simulink model "EngDem_TrqLimCoord"  (R2018a)
settings: configuration reference "cs_ert" (kept outside this file)
model workspace (MAT data in the model file):
  EngDem_TrqLimCoord_DT = 10
values from neighbouring files (symbols this model uses):
  EngDem_facAdj_C = 1.0    [EngDem_TrqLimCoord.sldd]
  EngDem_facAdjMax_C = 1.0    [EngDem_TrqLimCoord.sldd]
  EngDem_facAdjMin_C = 1.0    [EngDem_TrqLimCoord.sldd]
  EngDem_facDvolPT1_C = 50.0    [EngDem_TrqLimCoord.sldd]
  EngDem_facResFlowPT1_C = 50.0    [EngDem_TrqLimCoord.sldd]
  EngDem_RmpLimErrNeg_C = 50.0    [EngDem_TrqLimCoord.sldd]
  EngDem_RmpLimErrPos_C = 50.0    [EngDem_TrqLimCoord.sldd]
  EngDem_trqLimErr1_CUR : value not decoded    [EngDem_TrqLimCoord.sldd]
  EngDem_trqLimErr1_CURX : value not decoded    [EngDem_TrqLimCoord.sldd]
  EngDem_trqLimErr2_CUR : value not decoded    [EngDem_TrqLimCoord.sldd]
  EngDem_trqLimErr2_CURX : value not decoded    [EngDem_TrqLimCoord.sldd]
  EngDem_trqLimErr3_CUR : value not decoded    [EngDem_TrqLimCoord.sldd]
  EngDem_trqLimErr3_CURX : value not decoded    [EngDem_TrqLimCoord.sldd]
  EngDem_trqLimErr4_CUR : value not decoded    [EngDem_TrqLimCoord.sldd]
  EngDem_trqLimErr4_CURX : value not decoded    [EngDem_TrqLimCoord.sldd]
  EngDem_TrqLimErrRmpNeg_C = 50.0    [EngDem_TrqLimCoord.sldd]
  EngDem_TrqLimErrRmpPos_C = 100.0    [EngDem_TrqLimCoord.sldd]
  EngDem_trqLimPDiff_CUR : value not decoded    [EngDem_TrqLimCoord.sldd]
  EngDem_trqLimPDiff_CURX : value not decoded    [EngDem_TrqLimCoord.sldd]
undefined symbols (not defined in the file or in its folder): CEngDsT_tTransf_CURX, TRQ_MAX
libraries: sllib x4, simulink x2
settings Model: DataDictionary=EngDem_TrqLimCoord.sldd  Creator=zhoutinglin  LastModifiedBy=zhoutinglin

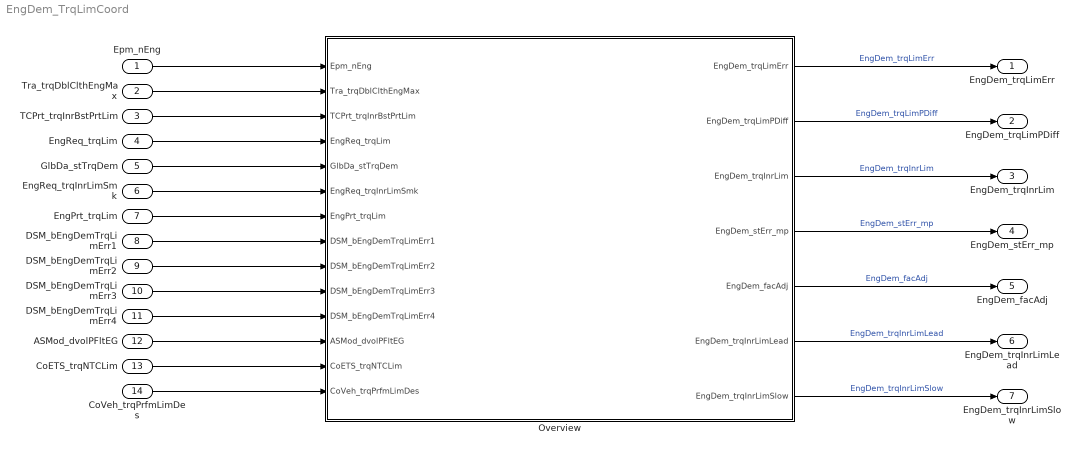
== system EngDem_TrqLimCoord ==
  Epm_nEng : Inport  Description=Engine speed  OutMin=0  OutMax=6000  OutDataTypeStr=ERPM  Unit=rpm  PortDimensions=[1 1]
  Tra_trqDblClthEngMax : Inport  Description=Application parameter for minimum torque of systemdegratation Nm  Port=2  OutMin=-3000  OutMax=3000  OutDataTypeStr=Torq  Unit=Nm  PortDimensions=[1 1]
  TCPrt_trqInrBstPrtLim : Inport  Description=Torque limitation from VGT Nm  Port=3  OutMin=-3276.8  OutMax=3276.7  OutDataTypeStr=Torq  Unit=Nm  PortDimensions=[1 1]
  EngReq_trqLim : Inport  Description=Resulting limiting torque from engine specifications  Port=4  OutMin=-3276.8  OutMax=3276.7  OutDataTypeStr=Torq  Unit=Nm  PortDimensions=[1 1]
  GlbDa_stTrqDem : Inport  Description=contains highest prior function with torque demand  Port=5  OutMin=0  OutMax=4294967295  OutDataTypeStr=State4  PortDimensions=[1 1]
  EngReq_trqInrLimSmk : Inport  Description=Limiting torque smoke limit  Port=6  OutMin=-3276.8  OutMax=3276.7  OutDataTypeStr=Torq  Unit=Nm  PortDimensions=[1 1]
  EngPrt_trqLim : Inport  Description=Limitation torque for engine mechanic protection by torque limitation (as inner engine torque)  Port=7  OutMin=-3276.8  OutMax=3276.7  OutDataTypeStr=Torq  Unit=Nm  PortDimensions=[1 1]
  DSM_bEngDemTrqLimErr1 : Inport  Description=FId for Engine demand Torque Limitation due to System error  Port=8  OutMin=0  OutMax=1  OutDataTypeStr=boolean  PortDimensions=[1 1]
  DSM_bEngDemTrqLimErr2 : Inport  Description=FId for Engine demand Torque Limitation due to System error  Port=9  OutMin=0  OutMax=1  OutDataTypeStr=boolean  PortDimensions=[1 1]
  DSM_bEngDemTrqLimErr3 : Inport  Description=FId for Engine demand Torque Limitation due to System error  Port=10  OutMin=0  OutMax=1  OutDataTypeStr=boolean  PortDimensions=[1 1]
  DSM_bEngDemTrqLimErr4 : Inport  Description=FId for Engine demand Torque Limitation due to System error  Port=11  OutMin=0  OutMax=1  OutDataTypeStr=boolean  PortDimensions=[1 1]
  ASMod_dvolPFltEG : Inport  Description=Calculated exhaust-gas volume flow in the particulate filter  Port=12  OutMin=0  OutMax=100  OutDataTypeStr=vFlow_m3ph  Unit=m^3/h  PortDimensions=[1 1]
  CoETS_trqNTCLim : Inport  Description=NTC torque limitation (0 in braking, ramped to max in braked to fired  Port=13  OutMin=0  OutMax=1000  OutDataTypeStr=Torq  Unit=Nm  PortDimensions=[1 1]
  CoVeh_trqPrfmLimDes : Inport  Description=Torque limitation from performence limiter  Port=14  OutMin=-3000  OutMax=3276.7  OutDataTypeStr=Torq  Unit=Nm  PortDimensions=[1 1]
  Overview : Subsystem
  EngDem_trqLimErr : Outport
  EngDem_trqLimPDiff : Outport  Port=2
  EngDem_trqInrLim : Outport  Port=3
  EngDem_stErr_mp : Outport  Port=4
  EngDem_facAdj : Outport  Port=5
  EngDem_trqInrLimLead : Outport  Port=6
  EngDem_trqInrLimSlow : Outport  Port=7
  wires:
  Epm_nEng/1 -> Overview/1(Epm_nEng)
  Tra_trqDblClthEngMax/1 -> Overview/2(Tra_trqDblClthEngMax)
  TCPrt_trqInrBstPrtLim/1 -> Overview/3(TCPrt_trqInrBstPrtLim)
  EngReq_trqLim/1 -> Overview/4(EngReq_trqLim)
  GlbDa_stTrqDem/1 -> Overview/5(GlbDa_stTrqDem)
  EngReq_trqInrLimSmk/1 -> Overview/6(EngReq_trqInrLimSmk)
  EngPrt_trqLim/1 -> Overview/7(EngPrt_trqLim)
  DSM_bEngDemTrqLimErr1/1 -> Overview/8(DSM_bEngDemTrqLimErr1)
  DSM_bEngDemTrqLimErr2/1 -> Overview/9(DSM_bEngDemTrqLimErr2)
  DSM_bEngDemTrqLimErr3/1 -> Overview/10(DSM_bEngDemTrqLimErr3)
  DSM_bEngDemTrqLimErr4/1 -> Overview/11(DSM_bEngDemTrqLimErr4)
  ASMod_dvolPFltEG/1 -> Overview/12(ASMod_dvolPFltEG)
  CoETS_trqNTCLim/1 -> Overview/13(CoETS_trqNTCLim)
  CoVeh_trqPrfmLimDes/1 -> Overview/14(CoVeh_trqPrfmLimDes)
  Overview/1(EngDem_trqLimErr) -> EngDem_trqLimErr/1  "EngDem_trqLimErr"
  Overview/2(EngDem_trqLimPDiff) -> EngDem_trqLimPDiff/1  "EngDem_trqLimPDiff"
  Overview/3(EngDem_trqInrLim) -> EngDem_trqInrLim/1  "EngDem_trqInrLim"
  Overview/4(EngDem_stErr_mp) -> EngDem_stErr_mp/1  "EngDem_stErr_mp"
  Overview/5(EngDem_facAdj) -> EngDem_facAdj/1  "EngDem_facAdj"
  Overview/6(EngDem_trqInrLimLead) -> EngDem_trqInrLimLead/1  "EngDem_trqInrLimLead"
  Overview/7(EngDem_trqInrLimSlow) -> EngDem_trqInrLimSlow/1  "EngDem_trqInrLimSlow"

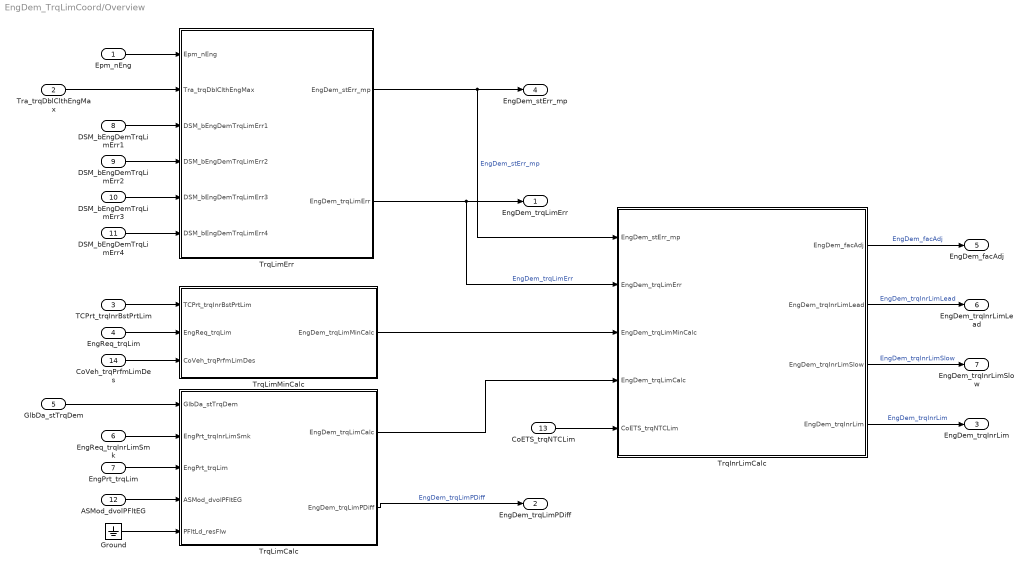
== system EngDem_TrqLimCoord/Overview ==
  Epm_nEng : Inport  Tag=rpm  Description=Engine speed  OutMin=0  OutMax=6000
  Tra_trqDblClthEngMax : Inport  Tag=Nm  Description=Application parameter for minimum torque of systemdegratation Nm  Port=2  OutMin=-3000  OutMax=3000
  TCPrt_trqInrBstPrtLim : Inport  Tag=Nm  Description=Torque limitation from VGT Nm  Port=3  OutMin=-3276.8  OutMax=3276.7
  EngReq_trqLim : Inport  Tag=Nm  Description=Resulting limiting torque from engine specifications  Port=4  OutMin=-3276.8  OutMax=3276.7
  GlbDa_stTrqDem : Inport  Description=contains highest prior function with torque demand  Port=5  OutMin=0  OutMax=4294967295
  EngReq_trqInrLimSmk : Inport  Tag=Nm  Description=Limiting torque smoke limit  Port=6  OutMin=-3276.8  OutMax=3276.7
  EngPrt_trqLim : Inport  Tag=Nm  Description=Limitation torque for engine mechanic protection by torque limitation (as inner engine torque)  Port=7  OutMin=-3276.8  OutMax=3276.7
  DSM_bEngDemTrqLimErr1 : Inport  Description=FId for Engine demand Torque Limitation due to System error  Port=8  OutMin=0  OutMax=1  OutDataTypeStr=boolean
  DSM_bEngDemTrqLimErr2 : Inport  Description=FId for Engine demand Torque Limitation due to System error  Port=9  OutMin=0  OutMax=1  OutDataTypeStr=boolean
  DSM_bEngDemTrqLimErr3 : Inport  Description=FId for Engine demand Torque Limitation due to System error  Port=10  OutMin=0  OutMax=1  OutDataTypeStr=boolean
  DSM_bEngDemTrqLimErr4 : Inport  Description=FId for Engine demand Torque Limitation due to System error  Port=11  OutMin=0  OutMax=1  OutDataTypeStr=boolean
  ASMod_dvolPFltEG : Inport  Tag=m^3/h  Description=Calculated exhaust-gas volume flow in the particulate filter  Port=12  OutMin=0  OutMax=100
  CoETS_trqNTCLim : Inport  Tag=Nm  Description=NTC torque limitation (0 in braking, ramped to max in braked to fired  Port=13  OutMin=0  OutMax=1000
  CoVeh_trqPrfmLimDes : Inport  Tag=Nm  Description=Torque limitation from performence limiter  Port=14  OutMin=-3000  OutMax=3276.7
  Ground : Ground
  TrqInrLimCalc : Subsystem
  TrqLimCalc : Subsystem  RTWFcnName=TrqLimCalc_Co  RTWFileName=TrqLimCalc
      settings: RTWSystemCode=Nonreusable function  RTWFcnNameOpts=User specified  RTWFileNameOpts=User specified
  TrqLimErr : Subsystem  RTWFcnName=TrqLimErr_Co  RTWFileName=TrqLimErr
      settings: RTWSystemCode=Nonreusable function  RTWFcnNameOpts=User specified  RTWFileNameOpts=User specified
  TrqLimMinCalc : Subsystem  RTWFcnName=TrqLimMinCalc_Co  RTWFileName=TrqLimMinCalc
      settings: RTWSystemCode=Nonreusable function  RTWFcnNameOpts=User specified  RTWFileNameOpts=User specified
  EngDem_trqLimErr : Outport  Tag=Nm  Description=Substitute limiting torque in the event of an error  OutMin=-3276.8  OutMax=3276.7
  EngDem_trqLimPDiff : Outport  Tag=Nm  Description=Limiting torque due to exhaust gas back-pressure  Port=2  OutMin=-3276.8  OutMax=3276.7
  EngDem_trqInrLim : Outport  Tag=Nm  Description=Resulting limiting torque (inner engine torque)  Port=3  OutMin=-3276.8  OutMax=3276.7
  EngDem_stErr_mp : Outport  Description=Status of the limitation FIDs  Port=4  OutMin=0  OutMax=1  OutDataTypeStr=boolean
  EngDem_facAdj : Outport  Description=EEPROM adjustment value for correction of the limiting torque  Port=5  OutMin=-10  OutMax=10
  EngDem_trqInrLimLead : Outport  Tag=Nm  Description=inner engine limted lead torque  Port=6  OutMin=-3276.8  OutMax=3276.7
  EngDem_trqInrLimSlow : Outport  Tag=Nm  Description=inner engine limted torque for Slow Path  Port=7  OutMin=-3276.8  OutMax=3276.7
  wires:
  Epm_nEng/1 -> TrqLimErr/1(Epm_nEng)
  TrqLimCalc/1(EngDem_trqLimCalc) -> TrqInrLimCalc/4(EngDem_trqLimCalc)
  CoETS_trqNTCLim/1 -> TrqInrLimCalc/5(CoETS_trqNTCLim)
  TrqInrLimCalc/2(EngDem_trqInrLimLead) -> EngDem_trqInrLimLead/1  "EngDem_trqInrLimLead"
  TrqLimCalc/2(EngDem_trqLimPDiff) -> EngDem_trqLimPDiff/1  "EngDem_trqLimPDiff"
  CoVeh_trqPrfmLimDes/1 -> TrqLimMinCalc/3(CoVeh_trqPrfmLimDes)
  DSM_bEngDemTrqLimErr3/1 -> TrqLimErr/5(DSM_bEngDemTrqLimErr3)
  Tra_trqDblClthEngMax/1 -> TrqLimErr/2(Tra_trqDblClthEngMax)
  TrqLimErr/2(EngDem_trqLimErr) -> EngDem_trqLimErr/1, TrqInrLimCalc/2(EngDem_trqLimErr)  "EngDem_trqLimErr"
  DSM_bEngDemTrqLimErr2/1 -> TrqLimErr/4(DSM_bEngDemTrqLimErr2)
  TrqLimMinCalc/1(EngDem_trqLimMinCalc) -> TrqInrLimCalc/3(EngDem_trqLimMinCalc)
  TrqInrLimCalc/3(EngDem_trqInrLimSlow) -> EngDem_trqInrLimSlow/1  "EngDem_trqInrLimSlow"
  TrqInrLimCalc/4(EngDem_trqInrLim) -> EngDem_trqInrLim/1  "EngDem_trqInrLim"
  DSM_bEngDemTrqLimErr4/1 -> TrqLimErr/6(DSM_bEngDemTrqLimErr4)
  TrqLimErr/1(EngDem_stErr_mp) -> EngDem_stErr_mp/1, TrqInrLimCalc/1(EngDem_stErr_mp)  "EngDem_stErr_mp"
  EngReq_trqLim/1 -> TrqLimMinCalc/2(EngReq_trqLim)
  EngPrt_trqLim/1 -> TrqLimCalc/3(EngPrt_trqLim)
  DSM_bEngDemTrqLimErr1/1 -> TrqLimErr/3(DSM_bEngDemTrqLimErr1)
  GlbDa_stTrqDem/1 -> TrqLimCalc/1(GlbDa_stTrqDem)
  TCPrt_trqInrBstPrtLim/1 -> TrqLimMinCalc/1(TCPrt_trqInrBstPrtLim)
  EngReq_trqInrLimSmk/1 -> TrqLimCalc/2(EngPrt_trqInrLimSmk)
  Ground/1 -> TrqLimCalc/5(PFltLd_resFlw)
  TrqInrLimCalc/1(EngDem_facAdj) -> EngDem_facAdj/1  "EngDem_facAdj"
  ASMod_dvolPFltEG/1 -> TrqLimCalc/4(ASMod_dvolPFltEG)

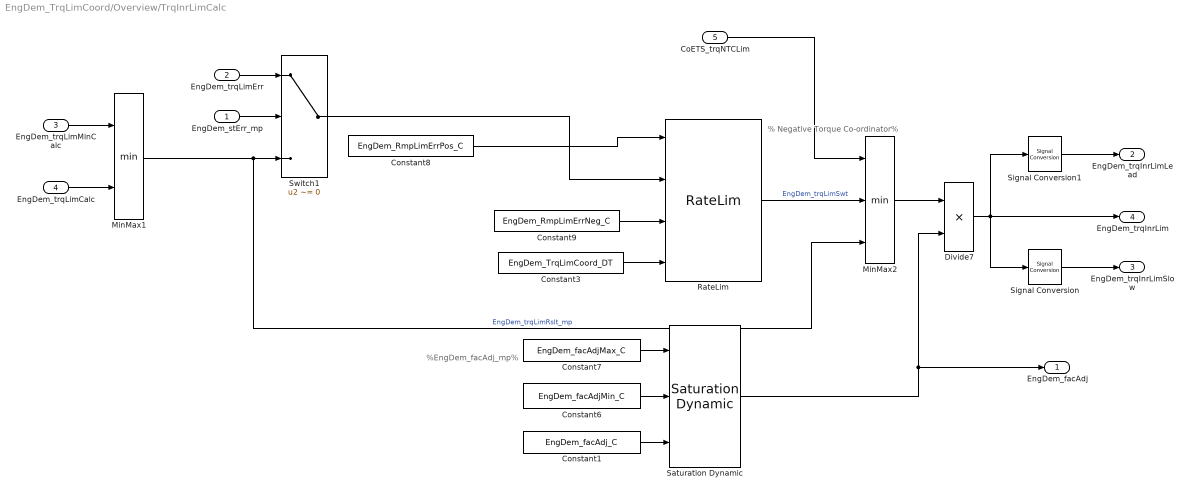
== system EngDem_TrqLimCoord/Overview/TrqInrLimCalc ==
  note: % Negative Torque Co-ordinator%
  note: %EngDem_facAdj_mp%
  EngDem_stErr_mp : Inport
  EngDem_trqLimErr : Inport  Port=2
  EngDem_trqLimMinCalc : Inport  Port=3
  EngDem_trqLimCalc : Inport  Port=4
  CoETS_trqNTCLim : Inport  Tag=Nm  Description=NTC torque limitation (0 in braking, ramped to max in braked to fired  Port=5
  Constant1 : Constant  Value=EngDem_facAdj_C
  Constant3 : Constant  Value=EngDem_TrqLimCoord_DT  OutDataTypeStr=Inherit: Inherit via back propagation
  Constant6 : Constant  Value=EngDem_facAdjMin_C
  Constant7 : Constant  Value=EngDem_facAdjMax_C
  Constant8 : Constant  Value=EngDem_RmpLimErrPos_C
  Constant9 : Constant  Value=EngDem_RmpLimErrNeg_C
  Divide7 : Product  Inputs=**  OutDataTypeStr=Inherit: Inherit via back propagation
  MinMax1 : MinMax  Inputs=2  InputSameDT=on
  MinMax2 : MinMax  Inputs=3  InputSameDT=on
  RateLim : sllib/RateLim
      settings: SourceProductName=sllib
  Saturation Dynamic : simulink/Discontinuities/Saturation Dynamic  OutMin=[]  OutMax=[]  OutDataTypeStr=Inherit: Same as second input  OutDataType=fixdt(1, 16)  OutScaling=2^-10  DoSatur=off
  Signal Conversion : SignalConversion  OverrideOpt=off
  Signal Conversion1 : SignalConversion  OverrideOpt=off
  Switch1 : Switch  Criteria=u2 ~= 0  InputSameDT=on
  EngDem_facAdj : Outport
  EngDem_trqInrLimLead : Outport  Port=2
  EngDem_trqInrLimSlow : Outport  Port=3
  EngDem_trqInrLim : Outport  Port=4
  wires:
  MinMax2/1 -> Divide7/1
  MinMax1/1 -> MinMax2/3, Switch1/3  "EngDem_trqLimRslt_mp"
  EngDem_trqLimCalc/1 -> MinMax1/2
  Constant1/1 -> Saturation Dynamic/3
  Constant6/1 -> Saturation Dynamic/2
  CoETS_trqNTCLim/1 -> MinMax2/1
  EngDem_trqLimMinCalc/1 -> MinMax1/1
  Constant7/1 -> Saturation Dynamic/1
  Saturation Dynamic/1 -> EngDem_facAdj/1, Divide7/2
  RateLim/1 -> MinMax2/2  "EngDem_trqLimSwt"
  Constant9/1 -> RateLim/3
  Constant8/1 -> RateLim/1
  Switch1/1 -> RateLim/2
  EngDem_trqLimErr/1 -> Switch1/1
  EngDem_stErr_mp/1 -> Switch1/2
  Constant3/1 -> RateLim/4
  Divide7/1 -> EngDem_trqInrLim/1, Signal Conversion/1, Signal Conversion1/1
  Signal Conversion1/1 -> EngDem_trqInrLimLead/1
  Signal Conversion/1 -> EngDem_trqInrLimSlow/1

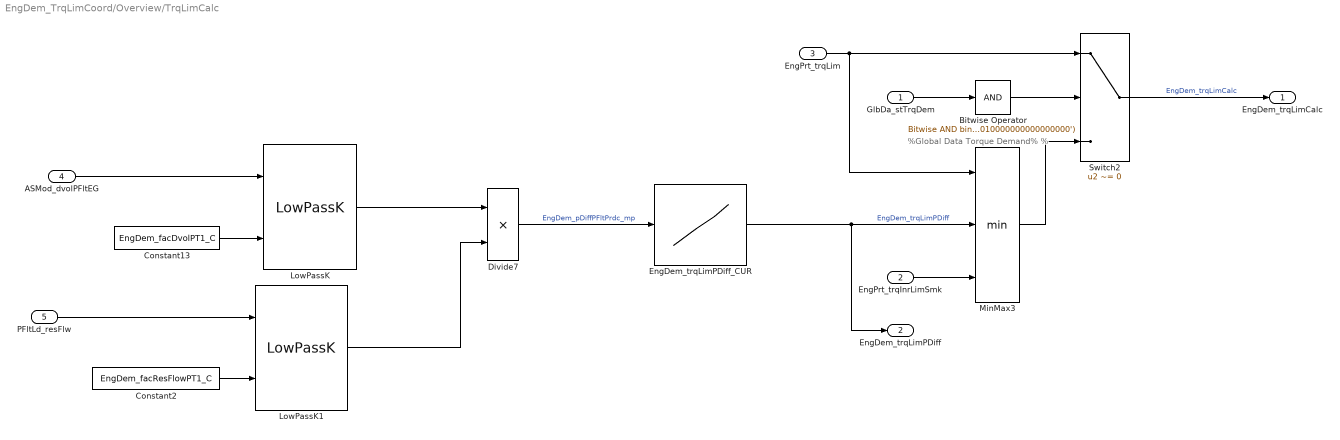
== system EngDem_TrqLimCoord/Overview/TrqLimCalc ==
  note: %Global Data Torque Demand% %
  GlbDa_stTrqDem : Inport
  EngPrt_trqInrLimSmk : Inport  Port=2
  EngPrt_trqLim : Inport  Port=3
  ASMod_dvolPFltEG : Inport  Tag=m^2/h  Description=Calculated exhaust-gas volume flow in the particulate filter  Port=4
  PFltLd_resFlw : Inport  Tag=kPa/(m^2/h)  Description=Flow resistance of the particulate filter  Port=5
  Bitwise Operator : simulink/Logic and Bit Operations/Bitwise Operator  logicop=AND  UseBitMask=on  BitMask=bin2dec('00000000000000010000000000000000')  BitMaskRealWorld=Stored Integer
  Constant13 : Constant  Value=EngDem_facDvolPT1_C
  Constant2 : Constant  Value=EngDem_facResFlowPT1_C
  Divide7 : Product  Inputs=**  OutDataTypeStr=Inherit: Inherit via back propagation
  EngDem_trqLimPDiff_CUR : Lookup_n-D  DialogController=Simulink.DDGSource  NumberOfTableDimensions=1  BreakpointsForDimension1=EngDem_trqLimPDiff_CURX  BreakpointsForDimension2=CEngDsT_tTransf_CURX  IndexSearchMethod=Linear search  BeginIndexSearchUsingPreviousIndexResult=on  Table=EngDem_trqLimPDiff_CUR  ExtrapMethod=Clip  UseLastTableValue=on  InternalRulePriority=Speed  OutDataTypeStr=Inherit: Inherit via back propagation  SaturateOnIntegerOverflow=on
  LowPassK : sllib/LowPassK
      settings: SourceProductName=sllib
  LowPassK1 : sllib/LowPassK
      settings: SourceProductName=sllib
  MinMax3 : MinMax  Inputs=3  InputSameDT=on
  Switch2 : Switch  Criteria=u2 ~= 0  InputSameDT=on
  EngDem_trqLimCalc : Outport
  EngDem_trqLimPDiff : Outport  Port=2
  wires:
  GlbDa_stTrqDem/1 -> Bitwise Operator/1
  EngPrt_trqLim/1 -> MinMax3/1, Switch2/1
  MinMax3/1 -> Switch2/3
  EngDem_trqLimPDiff_CUR/1 -> EngDem_trqLimPDiff/1, MinMax3/2  "EngDem_trqLimPDiff"
  Divide7/1 -> EngDem_trqLimPDiff_CUR/1  "EngDem_pDiffPFltPrdc_mp"
  ASMod_dvolPFltEG/1 -> LowPassK/1
  EngPrt_trqInrLimSmk/1 -> MinMax3/3
  Switch2/1 -> EngDem_trqLimCalc/1  "EngDem_trqLimCalc"
  Constant13/1 -> LowPassK/2
  Bitwise Operator/1 -> Switch2/2
  LowPassK1/1 -> Divide7/2
  LowPassK/1 -> Divide7/1
  Constant2/1 -> LowPassK1/2
  PFltLd_resFlw/1 -> LowPassK1/1

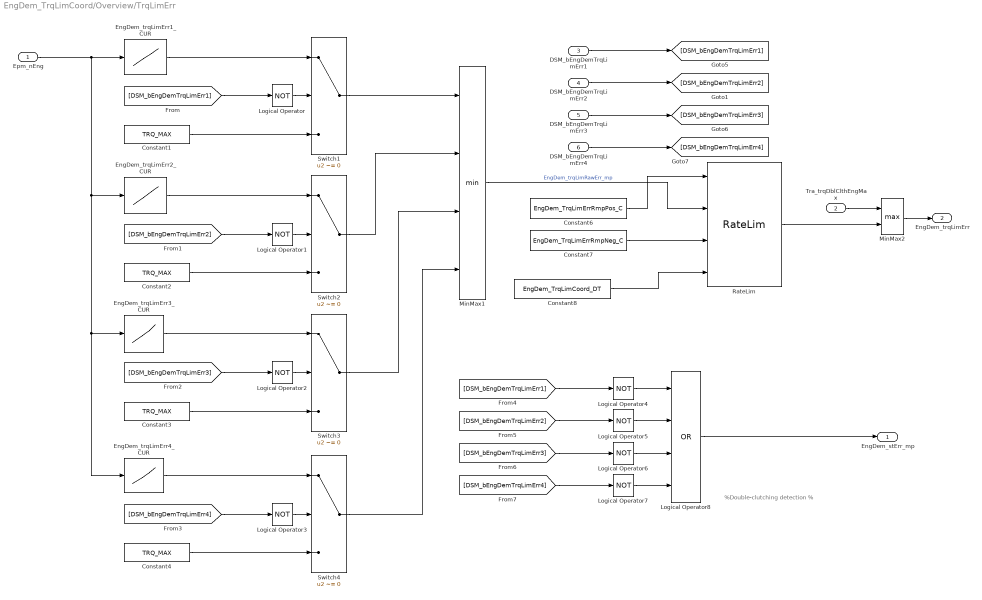
== system EngDem_TrqLimCoord/Overview/TrqLimErr ==
  note: %Double-clutching detection %
  Epm_nEng : Inport  Description=Engine speed
  Tra_trqDblClthEngMax : Inport  Port=2
  DSM_bEngDemTrqLimErr1 : Inport  Description=status of FId_EngDemTrqLimErr1  Port=3  OutMin=0  OutMax=1  OutDataTypeStr=boolean
  DSM_bEngDemTrqLimErr2 : Inport  Description=status of FId_EngDemTrqLimErr2  Port=4  OutMin=0  OutMax=1  OutDataTypeStr=boolean
  DSM_bEngDemTrqLimErr3 : Inport  Description=status of FId_EngDemTrqLimErr3  Port=5  OutMin=0  OutMax=1  OutDataTypeStr=boolean
  DSM_bEngDemTrqLimErr4 : Inport  Description=status of FId_EngDemTrqLimErr4  Port=6  OutMin=0  OutMax=1  OutDataTypeStr=boolean
  Constant{1..4} (4 alike) : Constant  Value=TRQ_MAX
  Constant6 : Constant  Value=EngDem_TrqLimErrRmpPos_C
  Constant7 : Constant  Value=EngDem_TrqLimErrRmpNeg_C
  Constant8 : Constant  Value=EngDem_TrqLimCoord_DT  OutDataTypeStr=Inherit: Inherit via back propagation
  EngDem_trqLimErr1_CUR : Lookup_n-D  DialogController=Simulink.DDGSource  NumberOfTableDimensions=1  BreakpointsForDimension1=EngDem_trqLimErr1_CURX  BreakpointsForDimension2=CEngDsT_tTransf_CURX  IndexSearchMethod=Linear search  BeginIndexSearchUsingPreviousIndexResult=on  Table=EngDem_trqLimErr1_CUR  ExtrapMethod=Clip  UseLastTableValue=on  InternalRulePriority=Speed  OutDataTypeStr=Inherit: Inherit via back propagation  SaturateOnIntegerOverflow=on
  EngDem_trqLimErr2_CUR : Lookup_n-D  DialogController=Simulink.DDGSource  NumberOfTableDimensions=1  BreakpointsForDimension1=EngDem_trqLimErr2_CURX  BreakpointsForDimension2=CEngDsT_tTransf_CURX  IndexSearchMethod=Linear search  BeginIndexSearchUsingPreviousIndexResult=on  Table=EngDem_trqLimErr2_CUR  ExtrapMethod=Clip  UseLastTableValue=on  InternalRulePriority=Speed  OutDataTypeStr=Inherit: Inherit via back propagation  SaturateOnIntegerOverflow=on
  EngDem_trqLimErr3_CUR : Lookup_n-D  DialogController=Simulink.DDGSource  NumberOfTableDimensions=1  BreakpointsForDimension1=EngDem_trqLimErr3_CURX  BreakpointsForDimension2=CEngDsT_tTransf_CURX  IndexSearchMethod=Linear search  BeginIndexSearchUsingPreviousIndexResult=on  Table=EngDem_trqLimErr3_CUR  ExtrapMethod=Clip  UseLastTableValue=on  InternalRulePriority=Speed  OutDataTypeStr=Inherit: Inherit via back propagation  SaturateOnIntegerOverflow=on
  EngDem_trqLimErr4_CUR : Lookup_n-D  DialogController=Simulink.DDGSource  NumberOfTableDimensions=1  BreakpointsForDimension1=EngDem_trqLimErr4_CURX  BreakpointsForDimension2=CEngDsT_tTransf_CURX  IndexSearchMethod=Linear search  BeginIndexSearchUsingPreviousIndexResult=on  Table=EngDem_trqLimErr4_CUR  ExtrapMethod=Clip  UseLastTableValue=on  InternalRulePriority=Speed  OutDataTypeStr=Inherit: Inherit via back propagation  SaturateOnIntegerOverflow=on
  Logical Operator{,1..7} (8 alike) : Logic  Operator=NOT  AllPortsSameDT=off  OutDataTypeStr=boolean
  Logical Operator8 : Logic  Operator=OR  Inputs=4  AllPortsSameDT=off  OutDataTypeStr=boolean
  MinMax1 : MinMax  Inputs=4  InputSameDT=on
  MinMax2 : MinMax  Function=max  Inputs=2  InputSameDT=on
  RateLim : sllib/RateLim
      settings: SourceProductName=sllib
  Switch{1..4} (4 alike) : Switch  Criteria=u2 ~= 0  InputSameDT=on
  EngDem_stErr_mp : Outport
  EngDem_trqLimErr : Outport  Port=2
  wires:
  MinMax1/1 -> RateLim/2  "EngDem_trqLimRawErr_mp"
  Switch1/1 -> MinMax1/1
  Logical Operator/1 -> Switch1/2
  [DSM_bEngDemTrqLimErr1] -> Logical Operator/1
  EngDem_trqLimErr1_CUR/1 -> Switch1/1
  Logical Operator1/1 -> Switch2/2
  [DSM_bEngDemTrqLimErr2] -> Logical Operator1/1
  EngDem_trqLimErr2_CUR/1 -> Switch2/1
  Switch2/1 -> MinMax1/2
  Logical Operator2/1 -> Switch3/2
  [DSM_bEngDemTrqLimErr3] -> Logical Operator2/1
  EngDem_trqLimErr3_CUR/1 -> Switch3/1
  Switch3/1 -> MinMax1/3
  Logical Operator3/1 -> Switch4/2
  [DSM_bEngDemTrqLimErr4] -> Logical Operator3/1
  EngDem_trqLimErr4_CUR/1 -> Switch4/1
  Switch4/1 -> MinMax1/4
  Epm_nEng/1 -> EngDem_trqLimErr4_CUR/1, EngDem_trqLimErr3_CUR/1, EngDem_trqLimErr2_CUR/1, EngDem_trqLimErr1_CUR/1
  Tra_trqDblClthEngMax/1 -> MinMax2/1
  Logical Operator4/1 -> Logical Operator8/1
  Logical Operator5/1 -> Logical Operator8/2
  Logical Operator6/1 -> Logical Operator8/3
  Logical Operator7/1 -> Logical Operator8/4
  Constant6/1 -> RateLim/1
  Constant7/1 -> RateLim/3
  RateLim/1 -> MinMax2/2
  Logical Operator8/1 -> EngDem_stErr_mp/1
  Constant1/1 -> Switch1/3
  Constant2/1 -> Switch2/3
  Constant3/1 -> Switch3/3
  Constant4/1 -> Switch4/3
  DSM_bEngDemTrqLimErr1/1 -> [DSM_bEngDemTrqLimErr1]
  DSM_bEngDemTrqLimErr2/1 -> [DSM_bEngDemTrqLimErr2]
  DSM_bEngDemTrqLimErr3/1 -> [DSM_bEngDemTrqLimErr3]
  DSM_bEngDemTrqLimErr4/1 -> [DSM_bEngDemTrqLimErr4]
  [DSM_bEngDemTrqLimErr1] -> Logical Operator4/1
  [DSM_bEngDemTrqLimErr2] -> Logical Operator5/1
  [DSM_bEngDemTrqLimErr3] -> Logical Operator6/1
  [DSM_bEngDemTrqLimErr4] -> Logical Operator7/1
  MinMax2/1 -> EngDem_trqLimErr/1
  Constant8/1 -> RateLim/4

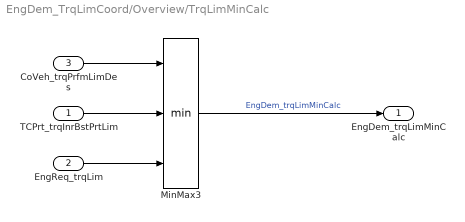
== system EngDem_TrqLimCoord/Overview/TrqLimMinCalc ==
  TCPrt_trqInrBstPrtLim : Inport
  EngReq_trqLim : Inport  Port=2
  CoVeh_trqPrfmLimDes : Inport  Tag=Nm  Description=Torque limitation from performence limiter  Port=3
  MinMax3 : MinMax  Inputs=3  InputSameDT=on
  EngDem_trqLimMinCalc : Outport
  wires:
  CoVeh_trqPrfmLimDes/1 -> MinMax3/1
  TCPrt_trqInrBstPrtLim/1 -> MinMax3/2
  EngReq_trqLim/1 -> MinMax3/3
  MinMax3/1 -> EngDem_trqLimMinCalc/1  "EngDem_trqLimMinCalc"
